simulink model "RX_ESP32"  (R2025b)
settings: Solver=FixedStepDiscrete  StartTime=0.0  StopTime=60  FixedStep=1.0  RelTol=1e-3  EnableMultiTasking=on
libraries: instrumentseriallib x2, svdutilitieslib x1
settings Model: ExtModeTrigDuration=2  Creator=daniel.camacho  LastModifiedBy=daniel.camacho
settings SolverCC: AutoInsertRateTranBlk=on
settings OptimizationCC: EnhancedBackFolding=on  PassReuseOutputArgsAs=Individual arguments  ZeroExternalMemoryAtStartup=off  ZeroInternalMemoryAtStartup=off  MaxStackSize=64  OptimizeBlockOrder=speed  DifferentSizesBufferReuse=on  OptimizationCustomize=off  EfficientTunableParamExpr=on
settings DebuggingCC: ParameterTunabilityLossMsg=error
settings HardwareCC: ProdBitPerPointer=32.0  ProdBitPerSizeT=32.0  ProdBitPerPtrDiffT=32.0  ProdLargestAtomicInteger=Long  ProdLargestAtomicFloat=Double  ProdWordSize=32.0  ProdHWDeviceType=ARM Compatible->ARM Cortex  UseEmbeddedCoderFeatures=off  UseSimulinkCoderFeatures=off
settings SFSimCC: MATLABDynamicMemAlloc=off
settings RTWCC: SystemTargetFile=ert.tlc  HardwareBoard=ESP32-WROVER (Arduino Compatible)  TLCOptions="-aInlineSetEventsForThisBaseRateFcn=TLC_FALSE -aSuppressMultiTaskScheduler=TLC_FALSE  -aRateBasedStepFcn=0"  TemplateMakefile=ert_default_tmf  Toolchain=ESP32  BuildConfiguration=Faster Runs  Description=Embedded Coder
settings CodeAppCC: ForceParamTrailComments=on  IgnoreCustomStorageClasses=off  OperatorAnnotations=on  SimulinkDataObjDesc=on  SFDataObjDesc=on  InsertBlockDesc=on
settings ERTTargetCC: ExtModeTransport=3.0  ExtModeStaticAlloc=on  ExtModeAutomaticAllocSize=off  ExtModeStaticAllocSize=65536.0  ExtModeMexFile=ext_xcp  ExtModeIntrfLevel=Level2 - Open  InlinedParameterPlacement=Hierarchical  SupportContinuousTime=on  SupportNonInlinedSFcns=on  SupportVariableSizeSignals=on

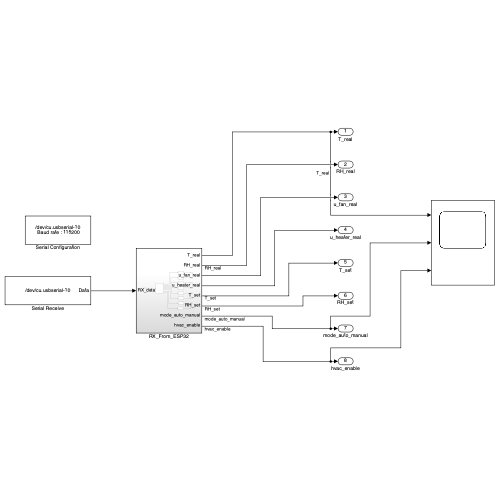
[thumbnail: Simulink's stored preview of the top-level diagram]
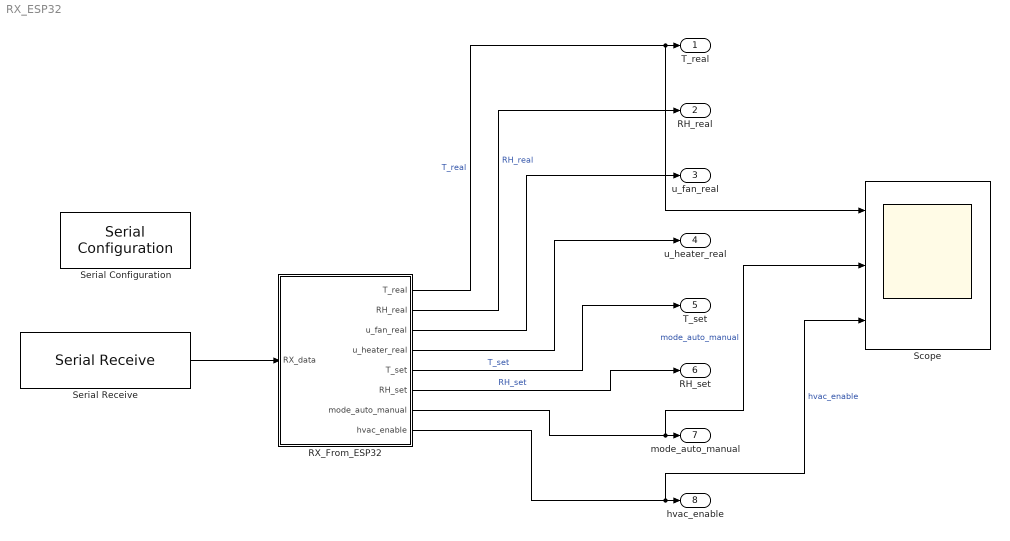
== system RX_ESP32 ==
  RX_From_ESP32 : Subsystem
  Scope : Scope  NumInputPorts=3
      settings: ActiveDisplayYMinimum=-1.8587351007590608E+16  ActiveDisplayYMaximum=9.885199254809798E+15
  Serial Configuration : instrumentseriallib/Serial Configuration  Priority=-200000  PortSel=/dev/cu.usbserial-10  Port=/dev/cu.usbserial-10  ComPort=/dev/cu.usbserial-10  BaudRate=115200  DataBits=8  Parity=none  StopBits=1  ByteOrder=little-endian  FlowControl=none  Timeout=10  SimulateUsing=Interpreted execution  BlockInModel=on  aMode=1
  Serial Receive : instrumentseriallib/Serial Receive  Priority=1  PortSel=/dev/cu.usbserial-10  Port=/dev/cu.usbserial-10  ComPort=/dev/cu.usbserial-10  DataType=uint8  SaveDataType=uint8  ToggleHeader=off  Header=[]  ToggleDataSize=on  DataSize=32  ToggleTerminator=off  Terminator=<none>  CustomTerminator=[]  InputFormat=Column major  EnableBlockingMode=on  ActionDataUnavailable=Output last received value  ActionWhenDataUnavailable=Output last received value  CustomValue=0  SampleTime=1  SimulateUsing=Interpreted execution  BlockInModel=on  aMode=1  LibraryInUse=instrumentlib
  T_real : Outport
  RH_real : Outport  Port=2
  u_fan_real : Outport  Port=3
  u_heater_real : Outport  Port=4
  T_set : Outport  Port=5
  RH_set : Outport  Port=6
  mode_auto_manual : Outport  Port=7
  hvac_enable : Outport  Port=8
  wires:
  RX_From_ESP32/4(u_heater_real) -> u_heater_real/1
  RX_From_ESP32/3(u_fan_real) -> u_fan_real/1
  RX_From_ESP32/6(RH_set) -> RH_set/1  "RH_set"
  RX_From_ESP32/2(RH_real) -> RH_real/1  "RH_real"
  RX_From_ESP32/1(T_real) -> Scope/1, T_real/1  "T_real"
  RX_From_ESP32/5(T_set) -> T_set/1  "T_set"
  Serial Receive/1 -> RX_From_ESP32/1(RX_data)
  RX_From_ESP32/7(mode_auto_manual) -> Scope/2, mode_auto_manual/1  "mode_auto_manual"
  RX_From_ESP32/8(hvac_enable) -> Scope/3, hvac_enable/1  "hvac_enable"

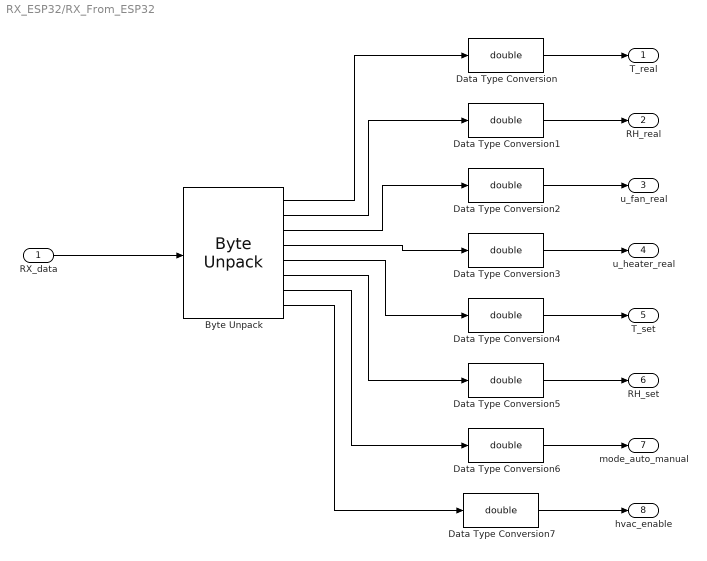
== system RX_ESP32/RX_From_ESP32 ==
  RX_data : Inport  OutDataTypeStr=uint8
  Byte Unpack : svdutilitieslib/Byte Unpack  dimensions={[1] [1] [1] [1] [1] [1] [1] [1]}  datatypes={'single','single','single','single','single','single','single','single'}  byteAlign=1  blockPlatform=arduinoert
  Data Type Conversion{,1..7} (8 alike) : DataTypeConversion  OutDataTypeStr=double  SaturateOnIntegerOverflow=off  RndMeth=Floor
  T_real : Outport
  RH_real : Outport  Port=2
  u_fan_real : Outport  Port=3
  u_heater_real : Outport  Port=4
  T_set : Outport  Port=5
  RH_set : Outport  Port=6
  mode_auto_manual : Outport  Port=7
  hvac_enable : Outport  Port=8
  wires:
  RX_data/1 -> Byte Unpack/1
  Byte Unpack/1 -> Data Type Conversion/1
  Byte Unpack/2 -> Data Type Conversion1/1
  Byte Unpack/3 -> Data Type Conversion2/1
  Byte Unpack/4 -> Data Type Conversion3/1
  Byte Unpack/5 -> Data Type Conversion4/1
  Byte Unpack/6 -> Data Type Conversion5/1
  Byte Unpack/7 -> Data Type Conversion6/1
  Byte Unpack/8 -> Data Type Conversion7/1
  Data Type Conversion/1 -> T_real/1
  Data Type Conversion1/1 -> RH_real/1
  Data Type Conversion2/1 -> u_fan_real/1
  Data Type Conversion3/1 -> u_heater_real/1
  Data Type Conversion4/1 -> T_set/1
  Data Type Conversion5/1 -> RH_set/1
  Data Type Conversion6/1 -> mode_auto_manual/1
  Data Type Conversion7/1 -> hvac_enable/1
